simulink subsystem "CSR"  (R2024b)
settings: Solver=VariableStepAuto  StartTime=0.0  StopTime=10.0  RelTol=1e-3
undefined symbols (not defined in the file): CSRInitialValue, SimuRISC_Constants
libraries: simulink x3
settings Model: Creator=stefano  LastModifiedBy=stefano

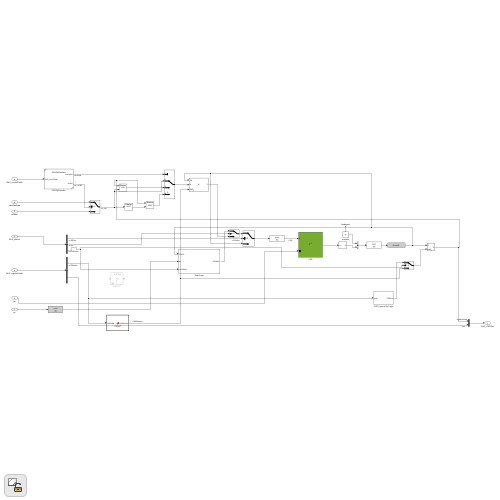
[thumbnail: Simulink's stored preview of the top-level diagram]
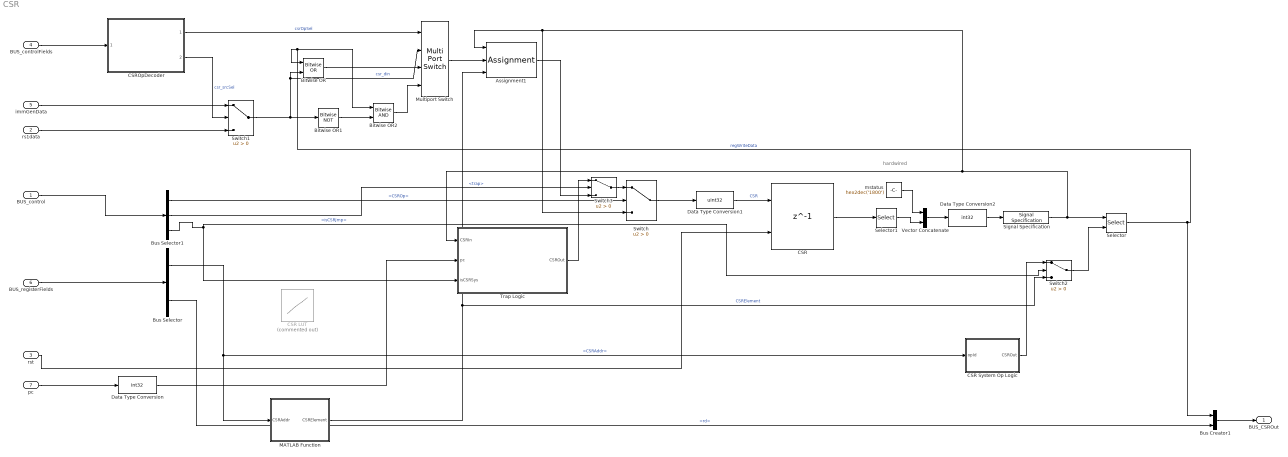
== system CSR ==
  note: hardwired
  BUS_control : Inport
  rs1data : Inport  Port=2
  rst : Inport  Port=3
  BUS_controlFields : Inport  Port=4
  immGenData : Inport  Port=5
  BUS_registerFields : Inport  Port=6
  pc : Inport  Port=7
  Assignment1 : Assignment  DiagnosticForDimensions=Warning  IndexOptions=Index vector (port)  Indices=1  OutputSizes=1
  Bitwise OR : simulink/Logic and Bit Operations/Bitwise Operator  logicop=OR  UseBitMask=off  NumInputPorts=2  BitMask=bin2dec('11011001')  BitMaskRealWorld=Stored Integer
      settings: LibrarySourceBlock=|
      | simulink/Quick Insert/Logic and Bit
      | Operations/Bitwise OR
  Bitwise OR1 : simulink/Logic and Bit Operations/Bitwise Operator  logicop=NOT  UseBitMask=off  BitMask=bin2dec('11011001')  BitMaskRealWorld=Stored Integer
      settings: LibrarySourceBlock=|
      | simulink/Quick Insert/Logic and Bit
      | Operations/Bitwise OR
  Bitwise OR2 : simulink/Logic and Bit Operations/Bitwise Operator  logicop=AND  UseBitMask=off  NumInputPorts=2  BitMask=bin2dec('11011001')  BitMaskRealWorld=Stored Integer
      settings: LibrarySourceBlock=|
      | simulink/Quick Insert/Logic and Bit
      | Operations/Bitwise OR
  Bus Creator1 : BusCreator  Inputs=2
  Bus Selector : BusSelector  OutputSignals=CSRAddr,rd
  Bus Selector1 : BusSelector  OutputSignals=CSROp,trap,isCSRJmp
  CSR : Delay  DelayLength=1  InitialCondition=CSRInitialValue  ExternalReset=Level hold
      settings: InputPortMap=u0,r5
  CSR LUT : Lookup_n-D  Commented=on  NumberOfTableDimensions=1  BreakpointsForDimension1=SimuRISC_Constants.CSR_LUT(:, 1)  IndexSearchMethod=Evenly spaced points  Table=SimuRISC_Constants.CSR_LUT(:, 2)  InterpMethod=Flat  ExtrapMethod=Clip  InternalRulePriority=Speed  RndMeth=Simplest
  CSR System Op Logic : Subsystem
  CSROpDecoder : Subsystem  ReferencedSubsystem=CSROpDecoder
  Data Type Conversion : DataTypeConversion  OutDataTypeStr=int32  ConvertRealWorld=Stored Integer (SI)  SaturateOnIntegerOverflow=off  RndMeth=Floor
  Data Type Conversion1 : DataTypeConversion  OutDataTypeStr=uint32  ConvertRealWorld=Stored Integer (SI)  SaturateOnIntegerOverflow=off  RndMeth=Floor
  Data Type Conversion2 : DataTypeConversion  OutDataTypeStr=int32  ConvertRealWorld=Stored Integer (SI)  SaturateOnIntegerOverflow=off  RndMeth=Floor
  MATLAB Function : MATLAB Function  TreatAsAtomicUnit=on
  Multiport Switch : MultiPortSwitch  DataPortOrder=Zero-based contiguous  zeroidx=on  SaturateOnIntegerOverflow=off  InputSameDT=off
  Selector : Selector  InputPortWidth=size(SimuRISC_Constants.CSR_LUT, 1)  IndexOptions=Index vector (port)  Indices=[1 3]  OutputSizes=1
  Selector1 : Selector  InputPortWidth=numel(CSRInitialValue)  IndexOptions=Index vector (dialog)  Indices=2:numel(CSRInitialValue)  OutputSizes=1
  Signal Specification : SignalSpecification  OutDataTypeStr=int32
  Switch{,1..3} (4 alike) : Switch  Criteria=u2 > Threshold  SaturateOnIntegerOverflow=off  InputSameDT=off
  Trap Logic : Subsystem
  Vector Concatenate : Concatenate
  mstatus : Constant  Value=hex2dec('1800')  OutDataTypeStr=uint32  SampleTime=-1
  BUS_CSROut : Outport
  wires:
  CSR/1 -> Selector1/1
  rst/1 -> CSR/2
  BUS_controlFields/1 -> CSROpDecoder/1
  Assignment1/1 -> Switch3/3
  BUS_control/1 -> Bus Selector1/1
  CSROpDecoder/2 -> Switch1/2  "csr_srcSel"
  MATLAB Function/1(CSRElement) -> Assignment1/3, Switch2/3  "CSRElement"
  CSROpDecoder/1 -> Multiport Switch/1  "csrOpSel"
  Switch1/1 -> Bitwise OR1/1, Multiport Switch/2, Bitwise OR/2  "csr_din"
  rs1data/1 -> Switch1/3
  Bus Selector1/1 -> Switch/2  "<CSROp>"
  BUS_registerFields/1 -> Bus Selector/1
  Multiport Switch/1 -> Assignment1/2
  Bitwise OR/1 -> Multiport Switch/3
  Signal Specification/1 -> Selector/1, Switch/3, Assignment1/1, Trap Logic/1(CSRIn)
  Bitwise OR2/1 -> Multiport Switch/4
  Bitwise OR1/1 -> Bitwise OR2/2
  Bus Selector/1 -> CSR System Op Logic/1(opId), MATLAB Function/1(CSRAddr)  "<CSRAddr>"
  Switch/1 -> Data Type Conversion1/1
  Bus Selector1/2 -> Switch3/2  "<trap>"
  Trap Logic/1(CSROut) -> Switch3/1
  pc/1 -> Data Type Conversion/1
  Switch3/1 -> Switch/1
  Data Type Conversion/1 -> Trap Logic/2(pc)
  Bus Selector1/3 -> Switch2/2, Trap Logic/3(isCSRSys)  "<isCSRJmp>"
  Switch2/1 -> Selector/2
  immGenData/1 -> Switch1/1
  CSR System Op Logic/1(CSROut) -> Switch2/1
  Data Type Conversion1/1 -> CSR/1  "CSR"
  Data Type Conversion2/1 -> Signal Specification/1
  Selector1/1 -> Vector Concatenate/2
  mstatus/1 -> Vector Concatenate/1
  Vector Concatenate/1 -> Data Type Conversion2/1
  Selector/1 -> Bitwise OR2/1, Bitwise OR/1, Bus Creator1/1  "regWriteData"
  Bus Selector/2 -> Bus Creator1/2  "<rd>"
  Bus Creator1/1 -> BUS_CSROut/1

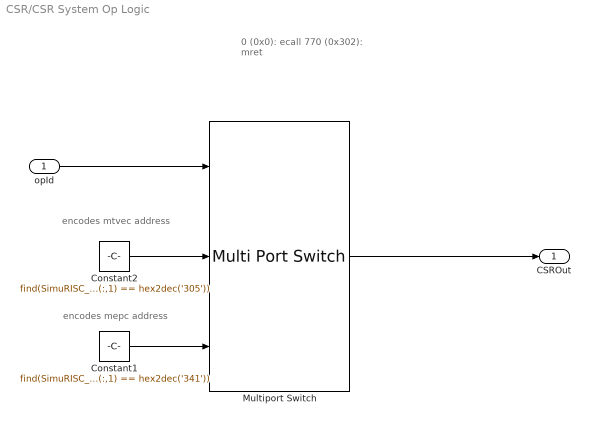
== system CSR/CSR System Op Logic ==
  note: encodes mtvec address
  note: encodes mepc address
  note: 0 (0x0): ecall
      | 770 (0x302): mret
  opId : Inport
  Constant1 : Constant  Value=find(SimuRISC_Constants.CSR_LUT(:,1) == hex2dec('341'))  OutDataTypeStr=int32  SampleTime=-1
  Constant2 : Constant  Value=find(SimuRISC_Constants.CSR_LUT(:,1) == hex2dec('305'))  OutDataTypeStr=int32  SampleTime=-1
  Multiport Switch : MultiPortSwitch  DataPortOrder=Specify indices  DataPortIndices={0, 770}  DiagnosticForDefault=None  SaturateOnIntegerOverflow=off  InputSameDT=off
  CSROut : Outport
  wires:
  Multiport Switch/1 -> CSROut/1
  Constant2/1 -> Multiport Switch/2
  opId/1 -> Multiport Switch/1
  Constant1/1 -> Multiport Switch/3

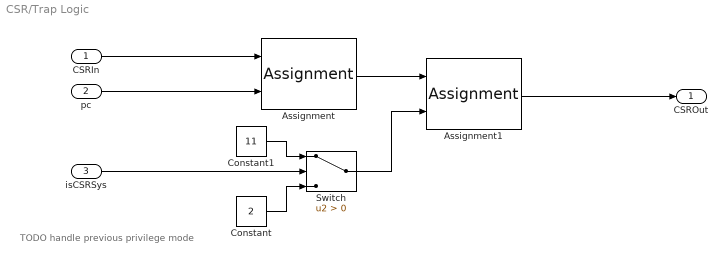
== system CSR/Trap Logic ==
  note: TODO handle previous privilege mode
  CSRIn : Inport
  pc : Inport  Port=2
  isCSRSys : Inport  Port=3
  Assignment : Assignment  DiagnosticForDimensions=Warning  IndexOptions=Index vector (dialog)  Indices=find(SimuRISC_Constants.CSR_LUT(:,1) == hex2dec('341'))  OutputSizes=1
  Assignment1 : Assignment  DiagnosticForDimensions=Warning  IndexOptions=Index vector (dialog)  Indices=find(SimuRISC_Constants.CSR_LUT(:,1) == hex2dec('342'))  OutputSizes=1
  Constant : Constant  Value=2  OutDataTypeStr=int32  SampleTime=-1
  Constant1 : Constant  Value=11  OutDataTypeStr=int32  SampleTime=-1
  Switch : Switch  Criteria=u2 > Threshold  SaturateOnIntegerOverflow=off  InputSameDT=off
  CSROut : Outport
  wires:
  Constant1/1 -> Switch/1
  Switch/1 -> Assignment1/2
  isCSRSys/1 -> Switch/2
  Constant/1 -> Switch/3
  Assignment/1 -> Assignment1/1
  pc/1 -> Assignment/2
  Assignment1/1 -> CSROut/1
  CSRIn/1 -> Assignment/1

== matlab function CSR/MATLAB Function ==
  data: CSRAddr input; CSRElement output
function CSRElement = CSRLUT(CSRAddr)
    CSRElement = int32(1);
    LUTBreakpoints = SimuRISC_Constants.CSR_LUT(:, 1);
    LUTElements = SimuRISC_Constants.CSR_LUT(:, 2);
    for iBP = 1:numel(LUTBreakpoints)
        if CSRAddr == LUTBreakpoints(iBP)
            CSRElement = LUTElements(iBP);
        end
    end
end
